simulink subsystem "OneMinusExpf"  (R2023b)
settings: Solver=VariableStepAuto  StartTime=0.0  StopTime=10.0  RelTol=1e-3
settings Model: Creator=dfurodet  LastModifiedBy=dfurodet

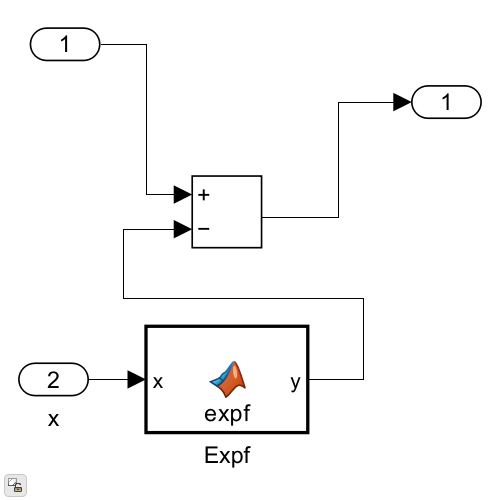
[thumbnail: Simulink's stored preview of the top-level diagram]
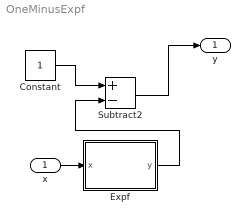
== system OneMinusExpf ==
  x : Inport
  Constant : Constant
  Expf : MATLAB Function  TreatAsAtomicUnit=on
  Subtract2 : Sum  Inputs=+-
  y : Outport
  wires:
  Expf/1(y) -> Subtract2/2
  Subtract2/1 -> y/1
  x/1 -> Expf/1(x)
  Constant/1 -> Subtract2/1

== matlab function OneMinusExpf/Expf ==
  data: x input; y output
function y = expf(x)
y = 1 + x / 1024;
y = y * y;
y = y * y;
y = y * y;
y = y * y;
y = y * y;
y = y * y;
y = y * y;
y = y * y;
y = y * y;
y = y * y;
